simulink model "RectifierThreePhases"  (R2020b)
settings: Solver=FixedStepAuto  StartTime=0.0  StopTime=0.1  FixedStep=Ts  RelTol=1e-3
InitFcn:
  | Ts=0.5e-3;
  | 
  | %Source Vac
  | Vs=230;
  | fs=50;
  | w=2*pi*fs;
  | Ls=300e-3;
  | 
  | Vcar=100;
libraries: powerlib x13
settings Model: Creator=SAGRIPANTI  LastModifiedBy=SAGRIPANTI

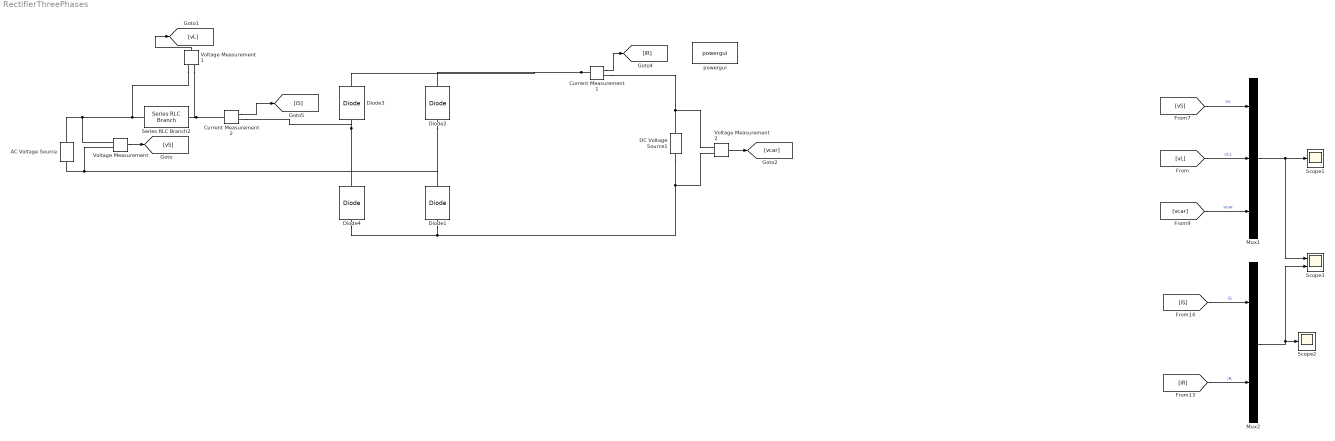
== system RectifierThreePhases ==
  AC Voltage Source : powerlib/Electrical Sources/AC Voltage Source  Amplitude=sqrt(2)*Vs  Phase=0  Frequency=fs  SampleTime=Ts  Measurements=None  BusType=swing  Pref=10e3  Qref=0  Qmin=-inf  Qmax=+inf
  Current Measurement1 : powerlib/Measurements/Current Measurement  PhasorSimulation=off  OutputType=Complex  PSBequivalent=0
  Current Measurement2 : powerlib/Measurements/Current Measurement  PhasorSimulation=off  OutputType=Complex  PSBequivalent=0
  DC Voltage Source1 : powerlib/Electrical Sources/DC Voltage Source  Amplitude=Vcar  Measurements=None
  Diode{1..4} (4 alike) : powerlib/Power Electronics/Diode  Ron=1e-6  Lon=0  Vf=0  IC=0  UseSnubber=0  Rs=500  Cs=250e-9  Measurements=off
  Mux1 : Mux  Inputs=3
  Mux2 : Mux  Inputs=2
  Scope1 : Scope
  Scope2 : Scope
  Scope3 : Scope  NumInputPorts=2
  Series RLC Branch2 : powerlib/Elements/Series RLC Branch  LConnTagsString=__new0  RConnTagsString=__new0  BranchType=L  Resistance=1e-6  Inductance=Ls  SetiL0=off  InitialCurrent=0  Capacitance=1e-6  Setx0=off  InitialVoltage=0  Measurements=None
  Voltage Measurement : powerlib/Measurements/Voltage Measurement  PhasorSimulation=off  OutputType=Complex  PSBequivalent=0
  Voltage Measurement1 : powerlib/Measurements/Voltage Measurement  PhasorSimulation=off  OutputType=Complex  PSBequivalent=0
  Voltage Measurement2 : powerlib/Measurements/Voltage Measurement  PhasorSimulation=off  OutputType=Complex  PSBequivalent=0
  powergui : powerlib/powergui  Priority=1  SimulationMode=Discrete  SampleTime=Ts  frequency=60  Iterations=50  frequencyindice=50  Pbase=100e6  ErrMax=1e-4  UnitsV=kV  UnitsW=MW  buscounter=0  FunctionMessages=off  echomessages=off  EnableUseOfTLC=off  CurrentSourceSwitches=off  DisableSnubberDevices=off  DisableRonSwitches=off  DisableVfSwitches=off  DisplayEquations=off  AutomaticDiscreteSolvers=off  SolverType=Tustin/Backward Euler (TBE)  Interpol=off  ExternalGateDelay=off  methode=off  Ts=100  x0status=blocks  SPID=on  SwTol=0  HookPort=off  NonlinearTolerance=1e-4  nMaxIteration=100  ContinueOnMaxIteration=off  RestoreLinks=warning  ResistiveCurrentMeasurement=off  Frange=[0:2:500]  Ylog=off  Xlog=on  ShowGrid=off  save=off  variable=ZData  structure=0  ZoomFFT=off  StartTime=0.0  cycles=1  DisplayStyle=1  fundamental=60  FreqAxis=off  MaxFrequency=1000  frequencyindicesteady=1  RmsSteady=1  display=off
  wires:
  Voltage Measurement/1 -> [vS]
  Current Measurement1/1 -> [iR]
  Voltage Measurement2/1 -> [vcar]
  Current Measurement2/1 -> [iS]
  [vS] -> Mux1/1  "Vs"
  Mux1/1 -> Scope3/1, Scope1/1
  [vL] -> Mux1/2  "vLs"
  [vcar] -> Mux1/3  "vcar"
  [iS] -> Mux2/1  "iS"
  [iR] -> Mux2/2  "iR"
  Mux2/1 -> Scope3/2, Scope2/1
  Voltage Measurement1/1 -> [vL]
  connections:
  Diode3/LConn1 -- Diode4/RConn1 -- Current Measurement2/RConn1
  Voltage Measurement/LConn2 -- Diode2/LConn1 -- Diode1/RConn1 -- AC Voltage Source/LConn1
  Current Measurement1/LConn1 -- Diode3/RConn1 -- Diode2/RConn1
  Current Measurement1/RConn1 -- DC Voltage Source1/RConn1 -- Voltage Measurement2/LConn1
  Diode4/LConn1 -- Diode1/LConn1 -- DC Voltage Source1/LConn1 -- Voltage Measurement2/LConn2
  AC Voltage Source/RConn1 -- Voltage Measurement/LConn1 -- Voltage Measurement1/LConn1 -- Series RLC Branch2/LConn1
  Series RLC Branch2/RConn1 -- Current Measurement2/LConn1 -- Voltage Measurement1/LConn2
